simulink model "Problem_3_Simulink"  (R2023a)
settings: Solver=FixedStepAuto  StartTime=0.0  StopTime=30  FixedStep=dt  RelTol=1e-3
values from neighbouring files (symbols this model uses):
  a = .1    (= 0.1)    [Problem_3_script.m]
  K = 10    [Problem_3_script.m]
  k_c = 2    [Problem_3_script.m]
  theta_0 = 0    [Problem_3_script.m]
  w = 3    [Problem_3_script.m]
  w_h = .1    (= 0.1)    [Problem_3_script.m]
  w_l = 1    [Problem_3_script.m]
  w_s = 10    [Problem_3_script.m]
  xi_s = 0.1    [Problem_3_script.m]
settings Model: Creator=eliasoa  LastModifiedBy=eliasoa

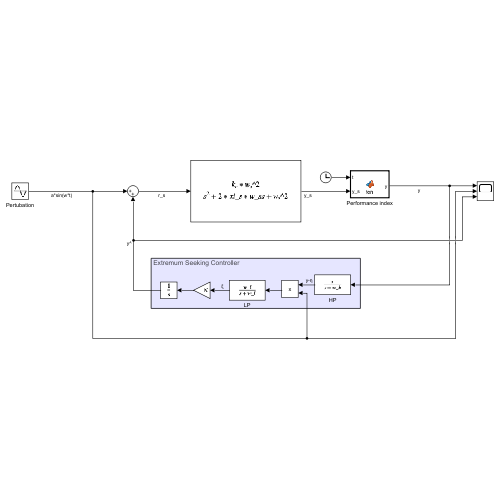
[thumbnail: Simulink's stored preview of the top-level diagram]
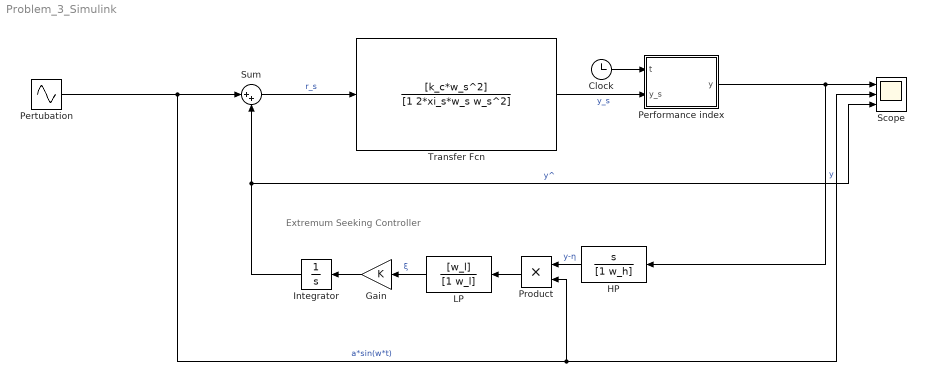
== system Problem_3_Simulink ==
  note: Extremum Seeking Controller
  Clock : Clock
  Gain : Gain  Gain=K
  HP : TransferFcn  Numerator=[1 0]  Denominator=[1 w_h]
  Integrator : Integrator  InitialCondition=theta_0
  LP : TransferFcn  Numerator=[w_l]  Denominator=[1 w_l]
  Performance index : MATLAB Function  TreatAsAtomicUnit=on
  Pertubation : Sin  Amplitude=a  Frequency=w  SampleTime=0
  Product : Product
  Scope : Scope  NumInputPorts=3
  Sum : Sum  Inputs=|++
  Transfer Fcn : TransferFcn  Numerator=[k_c*w_s^2]  Denominator=[1 2*xi_s*w_s w_s^2]
  wires:
  Integrator/1 -> Sum/2, Scope/3  "y^"
  LP/1 -> Gain/1  "ξ"
  Pertubation/1 -> Product/2, Scope/2, Sum/1  "a*sin(w*t)"
  Sum/1 -> Transfer Fcn/1  "r_s"
  Gain/1 -> Integrator/1
  Product/1 -> LP/1
  HP/1 -> Product/1  "y-η"
  Performance index/1(y) -> HP/1, Scope/1  "y"
  Transfer Fcn/1 -> Performance index/2(y_s)  "y_s"
  Clock/1 -> Performance index/1(t)

== matlab function Problem_3_Simulink/Performance index ==
  data: y output; t input; y_s input
function y = fcn(t,y_s)
y = -(0.5 - 0.1 * sin(0.01*t) - y_s)^2;
